simulink library "aerolibpropulsion2"  (Simulink 5.0)
libraries: simulink x3, aerolibatmos2 x1, aerolibasang x1, aerolibconvert x1
settings Model: Creator=sgage  LastModifiedBy=sgage  ExtModeAutoUpdateStatusClock=off

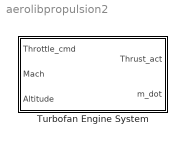
== system aerolibpropulsion2 ==
  Turbofan Engine System : Subsystem  mask(Turbofan Engine System){units=Metric (MKS), ic_source=Internal, IC=0, Fmax=45000, tau=1, SFC=0.35, Nt=0.9}
      mask prompts: ic_source "Initial thrust source:"; IC "Initial thrust:"; Fmax "Maximum sea-level static thrust:"; tau "Fastest engine time constant at sea-level static (sec):"; SFC "Sea-level static thrust specific fuel consumption:"; Nt "Ratio of installed thrust to uninstalled thrust:"
      mask help:
      | Implement a turbofan engine system. The turbofan engine system includes both engine and controller.
      |
      | Throttle position can vary from zero to one, corresponding to no to full throttle.  Altitude, initial thrust, and maximum thrust are entered in the same unit system as selected from the block for thrust and fuel flow output.
      mask init:
      | [ports,nondimT,nondimSFC, nondimTau] = aeroicon('aeroblkturbofan','icon');
      mask Help: web(asbhelp);
      mask StyleString: popup(Metric (MKS)|English),popup(Internal|External),edit,edit,edit,edit,edit
      mask CallbackString: aeroicon('aeroblkturbofan');|aeroicon('aeroblkturbofan');|||||
      mask Display:
      | port_label(ports(1).type,ports(1).port,ports(1).txt);
      | port_label(ports(2).type,ports(2).port,ports(2).txt);
      | port_label(ports(3).type,ports(3).port,ports(3).txt);
      | port_label(ports(4).type,ports(4).port,ports(4).txt);
      | port_label(ports(5).type,ports(5).port,ports(5).txt);
      | port_label(ports(6).type,ports(6).port,ports(6).txt);

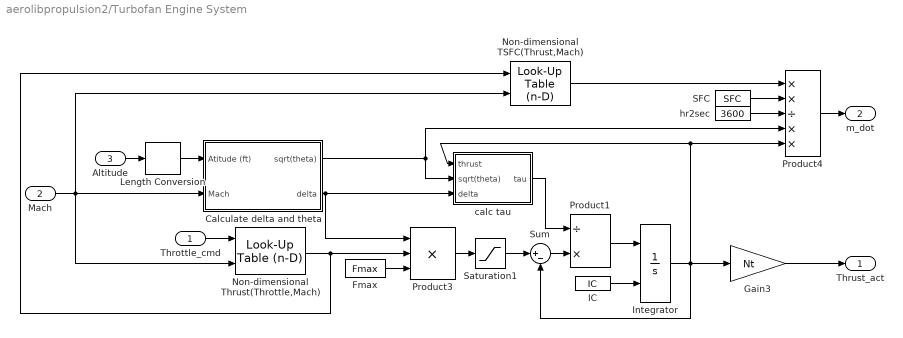
== system aerolibpropulsion2/Turbofan Engine System ==
  Throttle_cmd : Inport
  Mach : Inport  Port=2
  Altitude : Inport  Port=3
  Calculate delta and theta : Subsystem
  Fmax : Constant  Value=Fmax
  Gain3 : Gain  Gain=Nt  SaturateOnIntegerOverflow=on
  IC : Constant  Value=IC
  Integrator : Integrator  InitialConditionSource=external
  Length Conversion : aerolibconvert/Length Conversion  IU=m  OU=ft
  Non-dimensional TSFC(Thrust,Mach) : simulink/Look-Up Tables/Look-Up Table (n-D)  numDimsPopupSelect=2  bp1=[0.0:0.04:1.0]  bp2=[0:0.1:1.0]  bp3=[1:3]  bp4=[1:3]  bpcell={ [1:3], [1:3] }  explicitNumDims=2  searchMode=Linear Search  cacheBpFlag=on  vectorInputFlag=off  tableData=nondimSFC  interpMethod=Linear  extrapMethod=None - Clip  rangeErrorMode=Warning
  Non-dimensional Thrust(Throttle,Mach) : simulink/Look-Up Tables/Look-Up Table (n-D)  numDimsPopupSelect=2  bp1=[0 1]  bp2=[0:.1:1]  bp3=[0 1]  bp4=[1:3]  bpcell={ [1:3], [1:3] }  explicitNumDims=2  searchMode=Linear Search  cacheBpFlag=on  vectorInputFlag=off  tableData=nondimT  interpMethod=Linear  extrapMethod=None - Clip  rangeErrorMode=Warning
  Product1 : Product  Inputs=/*  SaturateOnIntegerOverflow=on  InputSameDT=on
  Product3 : Product  Inputs=3  SaturateOnIntegerOverflow=on  InputSameDT=on
  Product4 : Product  Inputs=**/**  SaturateOnIntegerOverflow=on  InputSameDT=on
  SFC : Constant  Value=SFC
  Saturation1 : Saturate  UpperLimit=Fmax  LowerLimit=0
  Sum : Sum  Inputs=|+-  SaturateOnIntegerOverflow=on  InputSameDT=on
  calc tau : Subsystem
  hr2sec : Constant  Value=3600
  Thrust_act : Outport
  m_dot : Outport  Port=2
  wires:
  Product4/1 -> m_dot/1
  calc tau/1(tau) -> Product1/1
  IC/1 -> Integrator/2
  Sum/1 -> Product1/2
  Product1/1 -> Integrator/1
  Integrator/1 -> Sum/2, Gain3/1, Product4/5, calc tau/1(thrust)
  Mach/1 -> Non-dimensional Thrust(Throttle,Mach)/2, Non-dimensional TSFC(Thrust,Mach)/2, Calculate delta and theta/2(Mach)
  Altitude/1 -> Length Conversion/1
  Throttle_cmd/1 -> Non-dimensional Thrust(Throttle,Mach)/1
  Length Conversion/1 -> Calculate delta and theta/1(Atitude (ft))
  Gain3/1 -> Thrust_act/1
  Calculate delta and theta/2("delta ") -> calc tau/3(delta), Product3/1
  Calculate delta and theta/1(sqrt(theta)) -> calc tau/2(sqrt(theta)), Product4/4
  Non-dimensional TSFC(Thrust,Mach)/1 -> Product4/1
  Product3/1 -> Saturation1/1
  Saturation1/1 -> Sum/1
  Non-dimensional Thrust(Throttle,Mach)/1 -> Product3/2, Non-dimensional TSFC(Thrust,Mach)/1
  hr2sec/1 -> Product4/3
  SFC/1 -> Product4/2
  Fmax/1 -> Product3/3

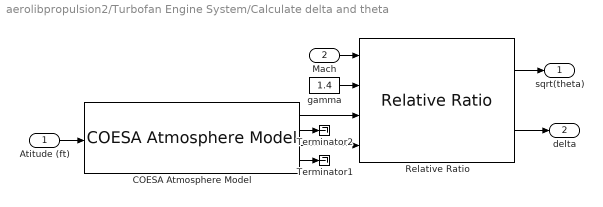
== system aerolibpropulsion2/Turbofan Engine System/Calculate delta and theta ==
  Atitude (ft) : Inport
  Mach : Inport  Port=2
  COESA Atmosphere Model : aerolibatmos2/COESA Atmosphere Model  units=English (Velocity in ft/s)  spec=1976 COESA-extended U.S. Standard Atmosphere  model=Profile  profile_var=High temperature  profile_percent=1%  profile_alt=5 km (16404 ft)  envelope_var=High temperature  envelope_percent=1%  action=Warning
  Relative Ratio : aerolibasang/Relative Ratio  units=English  theta=off  sq_theta=on  delta=on  sigma=off
  Terminator1 : Terminator
  Terminator2 : Terminator
  gamma : Constant  Value=1.4
  sqrt(theta) : Outport
  "delta " : Outport  Port=2
  wires:
  COESA Atmosphere Model/2 -> Terminator2/1
  COESA Atmosphere Model/4 -> Terminator1/1
  Relative Ratio/2 -> "delta "/1
  COESA Atmosphere Model/3 -> Relative Ratio/4
  Atitude (ft)/1 -> COESA Atmosphere Model/1
  Relative Ratio/1 -> sqrt(theta)/1
  COESA Atmosphere Model/1 -> Relative Ratio/3
  gamma/1 -> Relative Ratio/2
  Mach/1 -> Relative Ratio/1

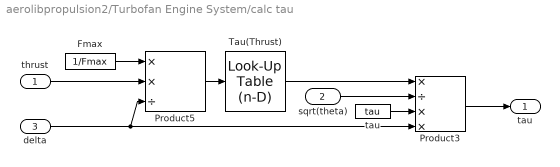
== system aerolibpropulsion2/Turbofan Engine System/calc tau ==
  thrust : Inport
  sqrt(theta) : Inport  Port=2
  delta : Inport  Port=3
  Fmax : Constant  Value=1/Fmax
  Product3 : Product  Inputs=*/**  SaturateOnIntegerOverflow=on  InputSameDT=on
  Product5 : Product  Inputs=**/  SaturateOnIntegerOverflow=on  InputSameDT=on
  Tau(Thrust) : simulink/Look-Up Tables/Look-Up Table (n-D)  numDimsPopupSelect=1  bp1=[0.0:0.04:1.0]  bp2=[10,22,31]  bp3=[1:3]  bp4=[1:3]  bpcell={ [1:3], [1:3] }  explicitNumDims=2  searchMode=Evenly Spaced Points  cacheBpFlag=off  vectorInputFlag=off  tableData=nondimTau  interpMethod=Linear  extrapMethod=None - Clip  rangeErrorMode=None
  "tau " : Constant  Value=tau
  tau : Outport
  wires:
  Product3/1 -> tau/1
  sqrt(theta)/1 -> Product3/2
  delta/1 -> Product3/4, Product5/3
  thrust/1 -> Product5/2
  Product5/1 -> Tau(Thrust)/1
  Tau(Thrust)/1 -> Product3/1
  "tau "/1 -> Product3/3
  Fmax/1 -> Product5/1
